simulink model "Sys2019"  (R2019a)
settings: Solver=ode45  StartTime=0.0  StopTime=.5  RelTol=1e-3  EnableMultiTasking=on
PreLoadFcn:
  | CONSTANTS
  | DEFAULT
  | Model
InitFcn:
  | CONSTANTS
  | DEFAULT
  | Model
values from neighbouring files (symbols this model uses):
  Amp0d = 1    [DEFAULT.m]    (also in Model.m = [0.25 8])
  Amp0n = 1    [DEFAULT.m]    (also in Model.m = [-3.125 -92])
  Amp1d = 1    [DEFAULT.m]    (also in Model.m = [0.25 8])
  Amp1n = 1    [DEFAULT.m]    (also in Model.m = [-3.125 -92])
  AmpSat0 = BIG    [DEFAULT.m]    (also in Model.m = 24)
  AmpSat1 = BIG    [DEFAULT.m]    (also in Model.m = 24)
  BackEMF0 = 0    [DEFAULT.m]    (also in Model.m = 0.0048)
  BackEMF1 = 0    [DEFAULT.m]    (also in Model.m = 0.0048)
  CtlSat0 = BIG    [DEFAULT.m]    (also in Model.m = 4.5)
  CtlSat1 = BIG    [DEFAULT.m]    (also in Model.m = 4.5)
  Elec0d = 1    [DEFAULT.m]    (also in Model.m = [0.0000873 1.13])
  Elec0n = 1    [DEFAULT.m]    (also in Model.m = [1])
  Elec1d = 1    [DEFAULT.m]    (also in Model.m = [0.0000873 1.13])
  Elec1n = 1    [DEFAULT.m]    (also in Model.m = [1])
  FB0 = 0    [DEFAULT.m]    (also in Model.m = 0.9)
  FB1 = 0    [DEFAULT.m]    (also in Model.m = 0.9)
  PID0 = [1 0 0]    [DEFAULT.m]    (also in Model.m = [-0.035 -0.003 -0.0097])
  PID1 = [1 0 0]    [DEFAULT.m]    (also in Model.m = [-0.035 -0.003 -0.0097])
  Sens0 = 1    [DEFAULT.m]    (also in Model.m = 1.1111)
  Sens1 = 1    [DEFAULT.m]    (also in Model.m = 1.1111)
  TConst0 = 1    [DEFAULT.m]    (also in Model.m = 0.0047)
  TConst1 = 1    [DEFAULT.m]    (also in Model.m = 0.0047)
libraries: simulink x6
settings Model: Creator=Leos  LastModifiedBy=K
settings DataIOCC: SaveFormat=Array  ReturnWorkspaceOutputs=off
settings OptimizationCC: ExpressionDepthLimit=2147483647  LifeSpan=inf
settings DebuggingCC: AlgebraicLoopMsg=none  UnderspecifiedInitializationDetection=Classic  MergeDetectMultiDrivingBlocksExec=none  SolverPrmCheckMsg=warning  FcnCallInpInsideContextMsg=warning  StateNameClashWarn=warning  SFUnexpectedBacktrackingDiag=warning  SFNoUnconditionalDefaultTransitionDiag=warning  SFExecutionAtInitializationDiag=none  ArithmeticOperatorsInVariantConditions=warning
settings HardwareCC: ProdBitPerPointer=32  ProdBitPerSizeT=32  ProdBitPerPtrDiffT=32  ProdLargestAtomicFloat=None  ProdIntDivRoundTo=Undefined  ProdEndianess=Unspecified  ProdWordSize=32  ProdHWDeviceType=32-bit Generic
settings ModelReferenceCC: PropagateSignalLabelsOutOfModel=off
settings SFSimCC: SimUseLocalCustomCode=off
settings RTWCC: RTWUseLocalCustomCode=off
settings CodeAppCC: StateflowObjectComments=on
settings GRTTargetCC: TargetLangStandard=C89/C90 (ANSI)  GeneratePreprocessorConditionals=Disable all  CombineOutputUpdateFcns=off  GRTInterface=on
settings ConfigComp: CovMetricSettings=dw  CovHtmlReporting=on  CovSaveCumulativeToWorkspaceVar=on  CovSaveSingleToWorkspaceVar=on  CovExternalEMLEnable=off  CovSFcnEnable=off
settings SimscapeCC: SimscapeNormalizeSystem=off

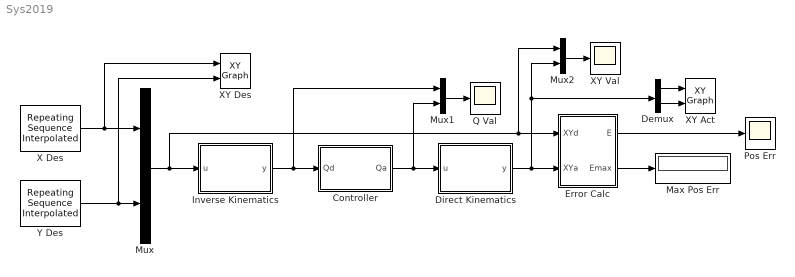
== system Sys2019 ==
  Controller : Subsystem
  Demux : Demux  Outputs=2
  Direct Kinematics : MATLAB Function  TreatAsAtomicUnit=on
  Error Calc : Subsystem
  Inverse Kinematics : MATLAB Function  TreatAsAtomicUnit=on
  Max Pos Err : Display
  Mux : Mux  Inputs=2
  Mux1 : Mux  Inputs=2
  Mux2 : Mux  Inputs=2
  Pos Err : Scope
  Q Val : Scope
  X Des : simulink/Sources/Repeating Sequence Interpolated  OutValues=Xd  TimeValues=Time  LookUpMeth=Interpolation-Use End Values  tsamp=SampleTime  OutMin=[]  OutMax=[]  OutDataTypeStr=double  OutputDataTypeScalingMode=double  OutDataType=fixdt(0,8)  OutScaling=2^-10
  XY Act : simulink/Sinks/XY Graph  xmin=-100  xmax=200  ymin=-100  ymax=200  st=-1
  XY Des : simulink/Sinks/XY Graph  xmin=-100  xmax=200  ymin=-100  ymax=200  st=-1
  XY Val : Scope
  Y Des : simulink/Sources/Repeating Sequence Interpolated  OutValues=Yd  TimeValues=Time  LookUpMeth=Interpolation-Use End Values  tsamp=SampleTime  OutMin=[]  OutMax=[]  OutDataTypeStr=double  OutputDataTypeScalingMode=double  OutDataType=fixdt(0,8)  OutScaling=2^-10
  wires:
  Y Des/1 -> XY Des/2, Mux/2
  X Des/1 -> XY Des/1, Mux/1
  Demux/2 -> XY Act/2
  Direct Kinematics/1(y) -> Mux2/2, Demux/1, Error Calc/2(XYa)
  Demux/1 -> XY Act/1
  Controller/1(Qa) -> Mux1/2, Direct Kinematics/1(u)
  Mux/1 -> Inverse Kinematics/1(u), Mux2/1, Error Calc/1(XYd)
  Error Calc/2(Emax) -> Max Pos Err/1
  Error Calc/1(E) -> Pos Err/1
  Inverse Kinematics/1(y) -> Mux1/1, Controller/1(Qd)
  Mux1/1 -> Q Val/1
  Mux2/1 -> XY Val/1

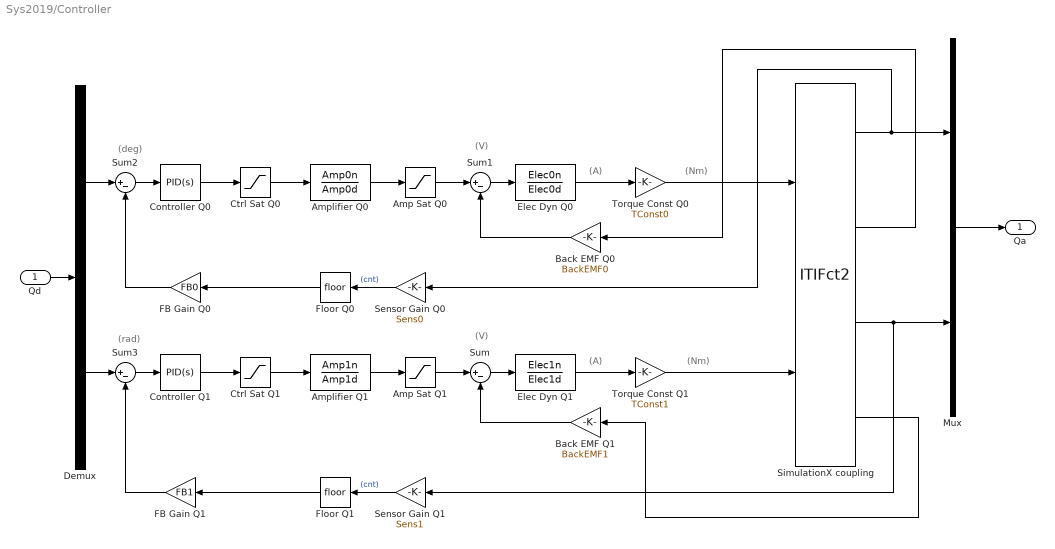
== system Sys2019/Controller ==
  note: (V)
  note: (rad)
  note: (A)
  note: (Nm)
  note: (V)
  note: (deg)
  note: (A)
  note: (Nm)
  Qd : Inport
  Amp Sat Q0 : Saturate  UpperLimit=AmpSat0  LowerLimit=-AmpSat0
  Amp Sat Q1 : Saturate  UpperLimit=AmpSat1  LowerLimit=-AmpSat1
  Amplifier Q0 : TransferFcn  Numerator=Amp0n  Denominator=Amp0d
  Amplifier Q1 : TransferFcn  Numerator=Amp1n  Denominator=Amp1d
  Back EMF Q0 : Gain  Gain=BackEMF0
  Back EMF Q1 : Gain  Gain=BackEMF1
  Controller Q0 : simulink/Continuous/PID Controller  Controller=PID  Form=Parallel  TimeDomain=Continuous-time  SampleTime=-1  IntegratorMethod=Forward Euler  FilterMethod=Forward Euler  ControllerParametersSource=internal  P=PID0(1)  I=PID0(2)  D=PID0(3)  UseFilter=on  N=100  TunerSelectOption=Transfer Function Based (PID Tuner App)  InitialConditionSource=internal  InitialConditionForIntegrator=0  InitialConditionForFilter=0  DifferentiatorICPrevScaledInput=0  ExternalReset=none  TrackingMode=off  Kt=1  LimitOutput=off  UpperSaturationLimit=inf  LowerSaturationLimit=-inf  LinearizeAsGain=on  AntiWindupMode=none  Kb=1  POutMin=[]  POutMax=[]  IOutMin=[]  IOutMax=[]  DOutMin=[]  DOutMax=[]  NOutMin=[]  NOutMax=[]  SumOutMin=[]  SumOutMax=[]  SaturationOutMin=[]  SaturationOutMax=[]  PParamMin=[]  PParamMax=[]  IParamMin=[]  IParamMax=[]  DParamMin=[]  DParamMax=[]  NParamMin=[]  NParamMax=[]  KbParamMin=[]  KbParamMax=[]  KtParamMin=[]  KtParamMax=[]  KbOutMin=[]  KbOutMax=[]  KtOutMin=[]  KtOutMax=[]  IntegratorOutMin=[]  IntegratorOutMax=[]  FilterOutMin=[]  FilterOutMax=[]  SumI1OutMin=[]  SumI1OutMax=[]  SumI2OutMin=[]  SumI2OutMax=[]  SumI3OutMin=[]  SumI3OutMax=[]  SumI4OutMin=[]  SumI4OutMax=[]  SumDOutMin=[]  SumDOutMax=[]  DifferentiatorOutMin=[]  DifferentiatorOutMax=[]  FilterDiffOutCoefMin=[]  FilterDiffOutCoefMax=[]  ReciprocalOutMin=[]  ReciprocalOutMax=[]  SumDenOutMin=[]  SumDenOutMax=[]  SumNumOutMin=[]  SumNumOutMax=[]  DivideOutMin=[]  DivideOutMax=[]  IntegratorContinuousStateAttributes=''  IntegratorStateMustResolveToSignalObject=off  IntegratorRTWStateStorageClass=Auto  FilterContinuousStateAttributes=''  FilterStateMustResolveToSignalObject=off  FilterRTWStateStorageClass=Auto  ParallelPVariant=InternalParameters  IdealPVariant=Disabled  IVariant=InternalParameters  DVariant=InternalParameters  IntegratorVariant=Continuous  SatVariant=Disabled  AWVariant=Passthrough  PCopyVariant=Disabled  TRVariant=Disabled  FdbkBlocksVariant=Forward  IdealPFdbkVariant=Disabled  SatFdbkVariant=Disabled  DerivativeFilterVariant=ContFilter  NVariant=InternalParameters  NCopyVariant=Disabled  FilterICVariant=InternalICsFilter  IntegratorICVariant=InternalICs  ExternalResetVariant=Disabled  TRSumVariant=Passthrough  SumFdbkVariant=Disabled  SumVariant=Sum_PID
  Controller Q1 : simulink/Continuous/PID Controller  Controller=PID  Form=Parallel  TimeDomain=Continuous-time  SampleTime=-1  IntegratorMethod=Forward Euler  FilterMethod=Forward Euler  ControllerParametersSource=internal  P=PID1(1)  I=PID1(2)  D=PID1(3)  UseFilter=on  N=100  TunerSelectOption=Transfer Function Based (PID Tuner App)  InitialConditionSource=internal  InitialConditionForIntegrator=0  InitialConditionForFilter=0  DifferentiatorICPrevScaledInput=0  ExternalReset=none  TrackingMode=off  Kt=1  LimitOutput=off  UpperSaturationLimit=inf  LowerSaturationLimit=-inf  LinearizeAsGain=on  AntiWindupMode=none  Kb=1  POutMin=[]  POutMax=[]  IOutMin=[]  IOutMax=[]  DOutMin=[]  DOutMax=[]  NOutMin=[]  NOutMax=[]  SumOutMin=[]  SumOutMax=[]  SaturationOutMin=[]  SaturationOutMax=[]  PParamMin=[]  PParamMax=[]  IParamMin=[]  IParamMax=[]  DParamMin=[]  DParamMax=[]  NParamMin=[]  NParamMax=[]  KbParamMin=[]  KbParamMax=[]  KtParamMin=[]  KtParamMax=[]  KbOutMin=[]  KbOutMax=[]  KtOutMin=[]  KtOutMax=[]  IntegratorOutMin=[]  IntegratorOutMax=[]  FilterOutMin=[]  FilterOutMax=[]  SumI1OutMin=[]  SumI1OutMax=[]  SumI2OutMin=[]  SumI2OutMax=[]  SumI3OutMin=[]  SumI3OutMax=[]  SumI4OutMin=[]  SumI4OutMax=[]  SumDOutMin=[]  SumDOutMax=[]  DifferentiatorOutMin=[]  DifferentiatorOutMax=[]  FilterDiffOutCoefMin=[]  FilterDiffOutCoefMax=[]  ReciprocalOutMin=[]  ReciprocalOutMax=[]  SumDenOutMin=[]  SumDenOutMax=[]  SumNumOutMin=[]  SumNumOutMax=[]  DivideOutMin=[]  DivideOutMax=[]  IntegratorContinuousStateAttributes=''  IntegratorStateMustResolveToSignalObject=off  IntegratorRTWStateStorageClass=Auto  FilterContinuousStateAttributes=''  FilterStateMustResolveToSignalObject=off  FilterRTWStateStorageClass=Auto  ParallelPVariant=InternalParameters  IdealPVariant=Disabled  IVariant=InternalParameters  DVariant=InternalParameters  IntegratorVariant=Continuous  SatVariant=Disabled  AWVariant=Passthrough  PCopyVariant=Disabled  TRVariant=Disabled  FdbkBlocksVariant=Forward  IdealPFdbkVariant=Disabled  SatFdbkVariant=Disabled  DerivativeFilterVariant=ContFilter  NVariant=InternalParameters  NCopyVariant=Disabled  FilterICVariant=InternalICsFilter  IntegratorICVariant=InternalICs  ExternalResetVariant=Disabled  TRSumVariant=Passthrough  SumFdbkVariant=Disabled  SumVariant=Sum_PID
  Ctrl Sat Q0 : Saturate  UpperLimit=CtlSat0  LowerLimit=-CtlSat0
  Ctrl Sat Q1 : Saturate  UpperLimit=CtlSat1  LowerLimit=-CtlSat1
  Demux : Demux  Outputs=2
  Elec Dyn Q0 : TransferFcn  Numerator=Elec0n  Denominator=Elec0d
  Elec Dyn Q1 : TransferFcn  Numerator=Elec1n  Denominator=Elec1d
  FB Gain Q0 : Gain  Gain=FB0
  FB Gain Q1 : Gain  Gain=FB1
  Floor Q0 : Rounding
  Floor Q1 : Rounding
  Mux : Mux  Inputs=2
  Sensor Gain Q0 : Gain  Gain=Sens0
  Sensor Gain Q1 : Gain  Gain=Sens1
  SimulationX coupling : S-Function  FunctionName=ITIFct2  Parameters=ip, port, ts, nIn, nOut  SFunctionDeploymentMode=off  EnableBusSupport=off  mask{ip='localhost', port=4097, ts=0.001, nIn=2, nOut=4}
      mask prompts: ip "Address: ip"; port "Port Number: port [-]"; ts "Communication Step Size: ts [s]"; nIn "Input Vector Dimension (to SimulationX): nIn [-]"; nOut "Output Vector Dimension (from SimulationX): nOut [-]"
      mask help: Coupling Element
  Sum{,1..3} (4 alike) : Sum  Inputs=|+-
  Torque Const Q0 : Gain  Gain=TConst0
  Torque Const Q1 : Gain  Gain=TConst1
  Qa : Outport
  wires:
  Qd/1 -> Demux/1
  Mux/1 -> Qa/1
  Sum/1 -> Elec Dyn Q1/1
  Sum3/1 -> Controller Q1/1
  Elec Dyn Q1/1 -> Torque Const Q1/1
  Amplifier Q1/1 -> Amp Sat Q1/1
  Amp Sat Q1/1 -> Sum/1
  Back EMF Q1/1 -> Sum/2
  Sum1/1 -> Elec Dyn Q0/1
  Sum2/1 -> Controller Q0/1
  Elec Dyn Q0/1 -> Torque Const Q0/1
  Amplifier Q0/1 -> Amp Sat Q0/1
  Amp Sat Q0/1 -> Sum1/1
  Back EMF Q0/1 -> Sum1/2
  Torque Const Q1/1 -> SimulationX coupling/2
  Demux/1 -> Sum2/1
  Demux/2 -> Sum3/1
  FB Gain Q0/1 -> Sum2/2
  FB Gain Q1/1 -> Sum3/2
  Torque Const Q0/1 -> SimulationX coupling/1
  Sensor Gain Q0/1 -> Floor Q0/1  "(cnt)"
  Floor Q0/1 -> FB Gain Q0/1
  Sensor Gain Q1/1 -> Floor Q1/1  "(cnt)"
  Floor Q1/1 -> FB Gain Q1/1
  Controller Q0/1 -> Ctrl Sat Q0/1
  Controller Q1/1 -> Ctrl Sat Q1/1
  Ctrl Sat Q0/1 -> Amplifier Q0/1
  Ctrl Sat Q1/1 -> Amplifier Q1/1
  SimulationX coupling/1 -> Sensor Gain Q0/1, Mux/1
  SimulationX coupling/3 -> Sensor Gain Q1/1, Mux/2
  SimulationX coupling/2 -> Back EMF Q0/1
  SimulationX coupling/4 -> Back EMF Q1/1

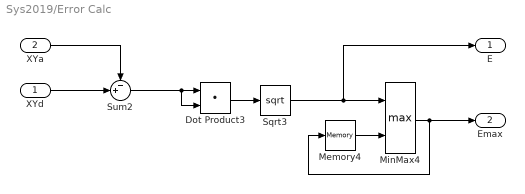
== system Sys2019/Error Calc ==
  XYd : Inport
  XYa : Inport  Port=2
  Dot Product3 : DotProduct  InputSameDT=on  OutDataTypeStr=Inherit: Inherit via internal rule
  Memory4 : Memory
  MinMax4 : MinMax  Function=max  Inputs=2
  Sqrt3 : Sqrt  SaturateOnIntegerOverflow=on
  Sum2 : Sum  Inputs=-+|
  E : Outport
  Emax : Outport  Port=2
  wires:
  XYa/1 -> Sum2/1
  Memory4/1 -> MinMax4/2
  MinMax4/1 -> Emax/1, Memory4/1
  XYd/1 -> Sum2/2
  Sum2/1 -> Dot Product3/2, Dot Product3/1
  Dot Product3/1 -> Sqrt3/1
  Sqrt3/1 -> E/1, MinMax4/1

== matlab function Sys2019/Direct Kinematics ==
  data: u input; y output
function y = DirKin(u)

theta_one = u(1);
theta_two = u(2);

theta_one = theta_one/-3;
theta_two = theta_two/-3;

coordinateX = 100*cosd(theta_one) + 100*cosd(theta_two);
coordinateY = 100*sind(theta_one) + 100*sind(theta_two);


% Return Default Result
y = [coordinateX;coordinateY];

== matlab function Sys2019/Inverse Kinematics ==
  data: u input; y output
function y = InvKin(u)

coordinateX = u(1);
coordinateY = u(2);

r = sqrt(coordinateX^2+coordinateY^2);
theta_d = atand(coordinateY/coordinateX);

theta_one = acosd(r/200)+ theta_d;
theta_two = 2*theta_d-theta_one;

theta_one = theta_one*-3;
theta_two = theta_two*-3;


% Return Default Result
y = [theta_one;theta_two];
